simulink model "BlueBird_RobotLocation"  (R2014a)
settings: Solver=FixedStepDiscrete  StartTime=0.0  StopTime=inf  FixedStep=0.033  RelTol=1e-3
undefined symbols (not defined in the file or in its folder): BlueBird_uni_todiff, simiam
libraries: KSim x2
settings Model: SnapshotBufferSize=100  Creator=jdelacroix  LastModifiedBy=Bird
settings DataIOCC: SignalLoggingSaveFormat=ModelDataLogs
settings OptimizationCC: ExpressionDepthLimit=2147483647
settings DebuggingCC: UnderspecifiedInitializationDetection=Classic  FcnCallInpInsideContextMsg=EnableAllAsWarning  StateNameClashWarn=warning

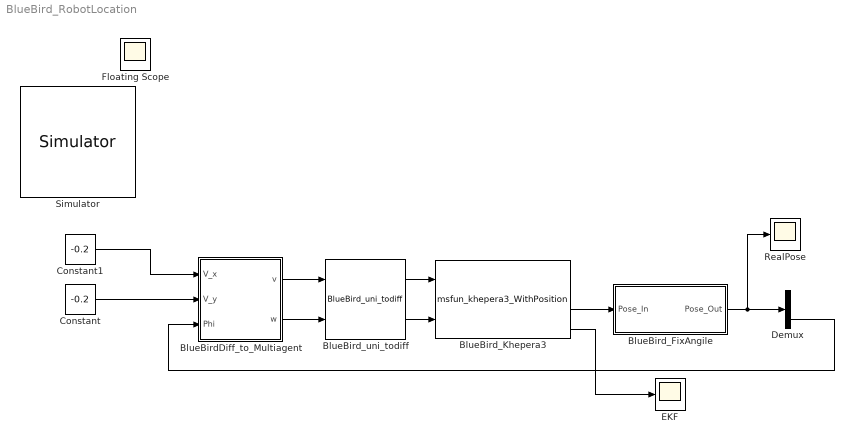
== system BlueBird_RobotLocation ==
  BlueBirdDiff_to_Multiagent : Subsystem  AncestorBlock=simiam/BlueBird_uni_todiff  mask(BlueBird_uni_todiff){l=2}
      mask prompts: l "偏移量（cm）"
      mask help: 这个模块完成自行车模型向机器人模型的转换。
  BlueBird_FixAngile : MATLAB Function  TreatAsAtomicUnit=on
  BlueBird_Khepera3 : M-S-Function  AncestorBlock=simiam/Khepera III  FunctionName=msfun_khepera3_WithPosition  Parameters=x_0,y_0,theta_0,ShowObservation  mask(Khepera3){x_0=0.1, y_0=0.1, theta_0=pi/2, robot_id=1, ShowObservation=on}
      mask prompts: robot_id "ID"; ShowObservation "显示观测"
      mask Display:
      | port_label('output', 1, 'ir_raw')
      | port_label('output', 2, 'wheel_ticks')
      | port_label('output', 3, 'PosFromSim')
      | port_label('output', 4, 'EKF_Out')
      | 
      | port_label('input', 1, 'vel_r')
      | port_label('input', 2, 'vel_l')
  BlueBird_uni_todiff : KSim/BlueBird_uni_todiff  r_R=0.021  r_L=0.021  b=0.0885
  Constant : Constant  Value=-0.2
  Constant1 : Constant  Value=-0.2
  Demux : Demux  Outputs=3
  EKF : Scope
      settings: YMin=-3.5  YMax=3.5  SaveName=ScopeData2
  RealPose : Scope
      settings: YMin=-3.5  YMax=3.5
  Simulator : KSim/Simulator  Priority=1
  Floating Scope : Scope
      settings: Floating=on
  wires:
  BlueBirdDiff_to_Multiagent/1(v) -> BlueBird_uni_todiff/1
  BlueBirdDiff_to_Multiagent/2(w) -> BlueBird_uni_todiff/2
  BlueBird_Khepera3/3 -> BlueBird_FixAngile/1(Pose_In)
  Constant/1 -> BlueBirdDiff_to_Multiagent/2(V_y)
  Constant1/1 -> BlueBirdDiff_to_Multiagent/1(V_x)
  Demux/3 -> BlueBirdDiff_to_Multiagent/3(Phi)
  BlueBird_uni_todiff/1 -> BlueBird_Khepera3/1
  BlueBird_uni_todiff/2 -> BlueBird_Khepera3/2
  BlueBird_Khepera3/4 -> EKF/1
  BlueBird_FixAngile/1(Pose_Out) -> RealPose/1, Demux/1

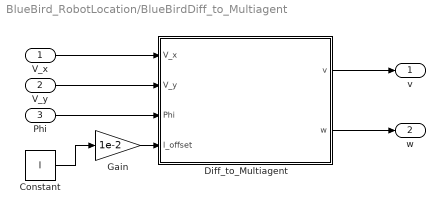
== system BlueBird_RobotLocation/BlueBirdDiff_to_Multiagent ==
  V_x : Inport
  V_y : Inport  Port=2
  Phi : Inport  Port=3
  Constant : Constant  Value=l
  Diff_to_Multiagent : MATLAB Function  TreatAsAtomicUnit=on
  Gain : Gain  Gain=1e-2
  v : Outport
  w : Outport  Port=2
  wires:
  V_x/1 -> Diff_to_Multiagent/1(V_x)
  V_y/1 -> Diff_to_Multiagent/2(V_y)
  Phi/1 -> Diff_to_Multiagent/3(Phi)
  Constant/1 -> Gain/1
  Gain/1 -> Diff_to_Multiagent/4(l_offset)
  Diff_to_Multiagent/1(v) -> v/1
  Diff_to_Multiagent/2(w) -> w/1

== matlab function BlueBird_RobotLocation/BlueBirdDiff_to_Multiagent/Diff_to_Multiagent ==
  data: V_x input; V_y input; v output; Phi input; l_offset input; w output
function [v,w] = BlueBird_Diff_to_Multiagent(V_x,V_y,Phi,l_offset)
%#codegen
%l_offset在这个函数里是米
if(l_offset >0)
    Temp = [1 0 ; 0 1/l_offset]*[cos(-Phi) -sin(-Phi); sin(-Phi) cos(-Phi)]*[V_x ; V_y];
    v = Temp(1,1);
    w = Temp(2,1);
else
    v = 0;
    w = 0;
end

== matlab function BlueBird_RobotLocation/BlueBird_FixAngile ==
  data: Pose_Out output; Pose_In input
function Pose_Out = FixAngile(Pose_In)
%用来修正过大的角度，输入域是：-pi-pi
Rad = Pose_In(3,1);
while (Rad > pi) 
    Rad = Rad - 2 * pi;
end
while (Rad < -pi) 
    Rad = Rad + 2 * pi;
end

Pose_Out = Pose_In;
Pose_Out(3,1) = Rad;
